simulink model "Push_pull_conv"  (R2021b)
settings: Solver=ode23s  StartTime=0.0  StopTime=inf  RelTol=1e-3
InitFcn:
  | % Target Load Voltage
  | v_ref = 48;
  | 
  | % Whether data should be broadcasted to Cloud / MQTT Ecosystem.
  | should_broadcast = true;
StartFcn:
  | if should_broadcast
  |     client = mqtt("tcp://rithviknishad.ddns.net");
  |     publish(client, "ps/state/IsRunning", "true");
  | end
StopFcn:
  | if should_broadcast
  |     client = mqtt("tcp://rithviknishad.ddns.net");
  |     publish(client, "ps/state/IsRunning", "false");
  | end
model workspace (MAT data in the model file):
  moreload = 1
undefined symbols (not defined in the file or in its folder): Ion, Lithium
libraries: spsSeriesRLCBranchLib x6, spsIdealSwitchLib x4, spsDiodeLib x4, spsMeanLib x3, simulink x3, spsCurrentMeasurementLib x2, spsGroundLib x2, spsMosfetLib x2, spsVariableResistorLib x1, slpidlib x1, spsPWMGeneratorDCDCLib x1, spsMultiWindingTransformerLib x1
(part 2 of 2)

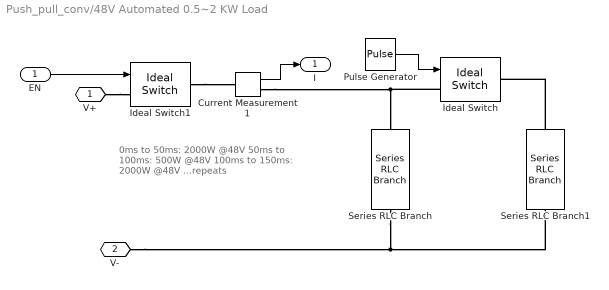
== system Push_pull_conv/48V Automated 0.5~2 KW Load ==
  note: 0ms to 50ms: 2000W @48V
      | 50ms to 100ms: 500W @48V
      | 100ms to 150ms: 2000W @48V
      | ...repeats
  EN : Inport
  Current Measurement1 : spsCurrentMeasurementLib/Current Measurement  PhasorSimulation=off  OutputType=Complex  PSBequivalent=0
  Ideal Switch : spsIdealSwitchLib/Ideal Switch  Ron=0.00000001  Lon=0  IC=0  Rs=1e5  Cs=inf  Measurements=off
  Ideal Switch1 : spsIdealSwitchLib/Ideal Switch  Ron=0.00000001  Lon=0  IC=0  Rs=1e5  Cs=inf  Measurements=off
  Pulse Generator : DiscretePulseGenerator  PulseType=Time based  Period=0.05  PulseWidth=50  PhaseDelay=0 * 0.1
  Series RLC Branch : spsSeriesRLCBranchLib/Series RLC Branch  LConnTagsString=__new0  RConnTagsString=__new0  BranchType=R  Resistance=48*48/500  Inductance=1e-3  SetiL0=off  InitialCurrent=0  Capacitance=41.42e-3  Setx0=off  InitialVoltage=0  Measurements=None
  Series RLC Branch1 : spsSeriesRLCBranchLib/Series RLC Branch  LConnTagsString=__new0  RConnTagsString=__new0  BranchType=R  Resistance=48*48/1500  Inductance=1e-3  SetiL0=off  InitialCurrent=0  Capacitance=41.42e-3  Setx0=off  InitialVoltage=0  Measurements=None
  V+ : PMIOPort  Side=Left
  V- : PMIOPort  Port=2  Side=Right
  I : Outport
  wires:
  Current Measurement1/1 -> I/1
  Pulse Generator/1 -> Ideal Switch/1
  EN/1 -> Ideal Switch1/1
  connections:
  Ideal Switch/LConn1 -- Series RLC Branch/LConn1 -- Current Measurement1/RConn1
  Series RLC Branch1/LConn1 -- Ideal Switch/RConn1
  Ideal Switch1/RConn1 -- Current Measurement1/LConn1
  Series RLC Branch1/RConn1 -- V-/RConn1 -- Series RLC Branch/RConn1
  V+/RConn1 -- Ideal Switch1/LConn1

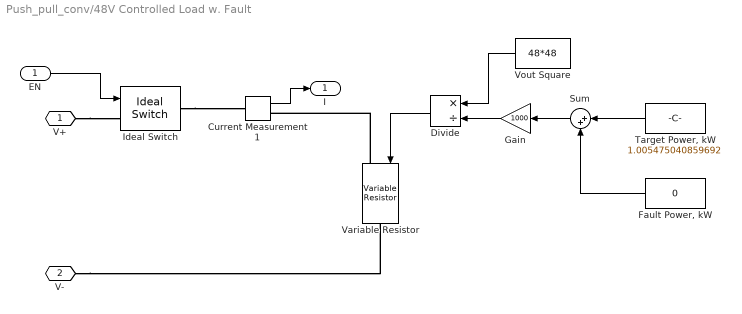
== system Push_pull_conv/48V Controlled Load w. Fault ==
  EN : Inport
  Current Measurement1 : spsCurrentMeasurementLib/Current Measurement  PhasorSimulation=off  OutputType=Complex  PSBequivalent=0
  Divide : Product  Inputs=*/
  "Fault Power, kW" : Constant  Value=0
  Gain : Gain  Gain=1000
  Ideal Switch : spsIdealSwitchLib/Ideal Switch  Ron=0.00000001  Lon=0  IC=0  Rs=1e5  Cs=inf  Measurements=off
  Sum : Sum  Inputs=|++
  "Target Power, kW" : Constant  Value=1.005475040859692
  Variable Resistor : spsVariableResistorLib/Variable Resistor  Rabsmin=1e-3
      settings: SourceProductBaseCode=PS
  Vout Square : Constant  Value=48*48
  V+ : PMIOPort  Side=Left
  V- : PMIOPort  Port=2  Side=Right
  I : Outport
  wires:
  Current Measurement1/1 -> I/1
  Vout Square/1 -> Divide/1
  Divide/1 -> Variable Resistor/1
  Gain/1 -> Divide/2
  EN/1 -> Ideal Switch/1
  "Target Power, kW"/1 -> Sum/1
  Sum/1 -> Gain/1
  "Fault Power, kW"/1 -> Sum/2
  connections:
  Ideal Switch/RConn1 -- Current Measurement1/LConn1
  Variable Resistor/LConn1 -- Current Measurement1/RConn1
  V+/RConn1 -- Ideal Switch/LConn1
  V-/RConn1 -- Variable Resistor/RConn1

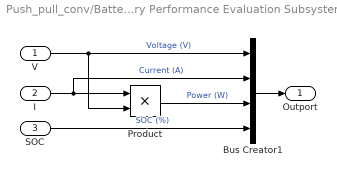
== system Push_pull_conv/Battery Performance Evaluation Subsystem ==
  V : Inport
  I : Inport  Port=2
  SOC : Inport  Port=3
  Bus Creator1 : BusCreator  Inputs=4
  Product : Product
  Outport : Outport
  wires:
  Bus Creator1/1 -> Outport/1
  I/1 -> Product/1, Bus Creator1/2  "Current (A)"
  V/1 -> Product/2, Bus Creator1/1  "Voltage (V)"
  Product/1 -> Bus Creator1/3  "Power (W)"
  SOC/1 -> Bus Creator1/4  "SOC (%)"

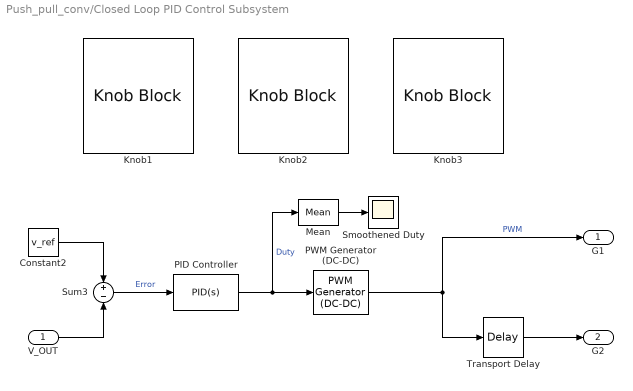
== system Push_pull_conv/Closed Loop PID Control Subsystem ==
  V_OUT : Inport
  Constant2 : Constant  Value=v_ref
  Knob1 : KnobBlock  LabelPosition=Bottom  ScaleMax=1  TickInterval=0.1
  Knob2 : KnobBlock  LabelPosition=Bottom  ScaleMax=1  TickInterval=0.1
  Knob3 : KnobBlock  LabelPosition=Bottom  ScaleMax=1  TickInterval=0.1
  Mean : spsMeanLib/Mean  Freq=150  Vinit=0  Ts=0
  PID Controller : slpidlib/PID Controller  Controller=PID  Form=Parallel  TimeDomain=Continuous-time  UseExternalTs=off  SampleTime=-1  IntegratorMethod=Forward Euler  FilterMethod=Forward Euler  ControllerParametersSource=internal  P=0.1  I=0.1  D=0  UseFilter=on  N=100  TunerSelectOption=Transfer Function Based (PID Tuner App)  InitialConditionSource=internal  InitialConditionForIntegrator=0  InitialConditionForFilter=0  DifferentiatorICPrevScaledInput=0  ExternalReset=none  TrackingMode=off  Kt=1  LimitOutput=on  SatLimitsSource=internal  UpperSaturationLimit=0.5  LowerSaturationLimit=0  LinearizeAsGain=off  AntiWindupMode=none  Kb=1  POutMin=[]  POutMax=[]  IOutMin=[]  IOutMax=[]  DOutMin=[]  DOutMax=[]  NOutMin=[]  NOutMax=[]  SumOutMin=[]  SumOutMax=[]  SaturationOutMin=[]  SaturationOutMax=[]  PParamMin=[]  PParamMax=[]  IParamMin=[]  IParamMax=[]  DParamMin=[]  DParamMax=[]  NParamMin=[]  NParamMax=[]  KbParamMin=[]  KbParamMax=[]  KtParamMin=[]  KtParamMax=[]  KbOutMin=[]  KbOutMax=[]  KtOutMin=[]  KtOutMax=[]  IntegratorOutMin=[]  IntegratorOutMax=[]  FilterOutMin=[]  FilterOutMax=[]  SumI1OutMin=[]  SumI1OutMax=[]  SumI2OutMin=[]  SumI2OutMax=[]  SumI3OutMin=[]  SumI3OutMax=[]  SumI4OutMin=[]  SumI4OutMax=[]  SumDOutMin=[]  SumDOutMax=[]  DifferentiatorOutMin=[]  DifferentiatorOutMax=[]  FilterDiffOutCoefMin=[]  FilterDiffOutCoefMax=[]  ReciprocalOutMin=[]  ReciprocalOutMax=[]  SumDenOutMin=[]  SumDenOutMax=[]  SumNumOutMin=[]  SumNumOutMax=[]  DivideOutMin=[]  DivideOutMax=[]  UdiffTsProdOutMin=[]  UdiffTsProdOutMax=[]  NTsProdOutMin=[]  NTsProdOutMax=[]  UintegralTsProdOutMin=[]  UintegralTsProdOutMax=[]  UngainTsProdOutMin=[]  UngainTsProdOutMax=[]  IntegratorContinuousStateAttributes=''  IntegratorStateMustResolveToSignalObject=off  IntegratorRTWStateStorageClass=Auto  FilterContinuousStateAttributes=''  FilterStateMustResolveToSignalObject=off  FilterRTWStateStorageClass=Auto  ParallelPVariant=InternalParameters  IdealPVariant=Disabled  IVariant=InternalParameters  DVariant=InternalParameters  IntegratorVariant=Continuous  SatVariant=Enabled  AWVariant=Passthrough  PCopyVariant=Disabled  TRVariant=Disabled  FdbkBlocksVariant=Forward  IdealPFdbkVariant=Disabled  SatFdbkVariant=Disabled  DerivativeFilterVariant=ContFilter  NVariant=InternalParameters  NCopyVariant=Disabled  FilterICVariant=InternalICsFilter  IntegratorICVariant=InternalICs  ExternalResetVariant=Disabled  TRSumVariant=Passthrough  SumFdbkVariant=Disabled  SumVariant=Sum_PID  TsampFilterVariant=InternalTs  TsampNgainVariant=Passthrough  TsampIntegralVariant=Passthrough  ExternalSaturationOutDataTypeStr=Inherit: Same as second input
  PWM Generator (DC-DC) : spsPWMGeneratorDCDCLib/PWM Generator (DC-DC)  Fsw=150e3  Ts=0
  Smoothened Duty : Scope
  Sum3 : Sum  Inputs=+-
  Transport Delay : TransportDelay  DelayTime=180/(360*150e3)
  G1 : Outport
  G2 : Outport  Port=2
  wires:
  Constant2/1 -> Sum3/1
  V_OUT/1 -> Sum3/2
  PWM Generator (DC-DC)/1 -> G1/1, Transport Delay/1  "PWM"
  Sum3/1 -> PID Controller/1  "Error"
  PID Controller/1 -> Mean/1, PWM Generator (DC-DC)/1  "Duty"
  Mean/1 -> Smoothened Duty/1
  Transport Delay/1 -> G2/1

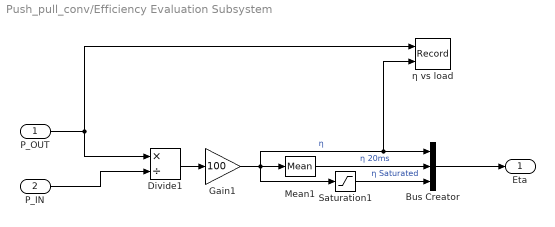
== system Push_pull_conv/Efficiency Evaluation Subsystem ==
  P_OUT : Inport
  P_IN : Inport  Port=2
  Bus Creator : BusCreator  Inputs=3
  Divide1 : Product  Inputs=*/
  Gain1 : Gain  Gain=100
  Mean1 : spsMeanLib/Mean  Freq=50  Vinit=0  Ts=0
  Saturation1 : Saturate  UpperLimit=100
  η vs load : Record  FileSettingsInternal="{\"entries\":[{\"content\":{\"excelSettings\":{\"content\":{},\"type\":\"Streamout.ExcelSettings\"}},\"type\":\"Streamout.FileSettingStorage\",\"uuid\":\"d06f74cc-fced-4a1e-9c31-17602b41e559\"}],\"packageUris\":[\"http://schema.mathworks.com/mf0/streamout_blocks/R2020a\"],\"version\":\"1.0\"}"  Layout=[1 1]  SignalsInternal="{\"entries\":[{\"content\":{\"signals\":[{\"content\":{\"blockPath\":[\"Push_pull_conv/Efficiency Evaluation Subsystem/η vs load\"],\"channel\":[],\"dimensions\":[1],\"domain\":\"Push_pull_conv/Efficiency Evaluation Subsystem/ￎﾷ vs load\",\"lineColor\":\"#64d413\",\"plots\":[],\"port\":1,\"sid\":[\"\"],\"signalID\":227180,\"signalName\":\"P_OUT\"},\"type\":\"RecordBlkView.Signal\",\"uuid\":\"f3186113-8e68-4c99-bf8f-1509c4a87657\"},{\"content\":{\"blockPath\":[\"Push_pull_conv/Efficiency Evaluation Subsystem/η vs load\"],\"channel\":[],\"dimensions\":[1],\"domain\":\"Push_pull_conv/Efficiency Evaluation Subsystem/ￎﾷ vs load\",\"lineColor\":\"#ff13a6\",\"plots\":[],\"port\":2,\"sid\":[\"\"],\"signalID\":227184,\"signalName\":\"η\"},\"type\":\"RecordBlkView.Signal\",\"uuid\":\"933036bb-5959-4669-957e-8a4b6c9fc7ee\"}]},\"type\":\"RecordBlkView.InputSignals\",\"uuid\":\"264eb576-88f5-4594-8ef1-38e7c656bcfb\"}],\"packageUris\":[\"http://schema.mathworks.com/mf0/streamout_blocks/R2020a\"],\"version\":\"1.0\"}"  VisualizationBindings="{\"xyplotplugin\":{\"info\":[{\"series\":[],\"subplotID\":1}]}}"  CompatibilityTag=XY
  Eta : Outport
  wires:
  Gain1/1 -> Saturation1/1, η vs load/2, Bus Creator/1, Mean1/1  "η"
  Saturation1/1 -> Bus Creator/3  "η Saturated"
  Divide1/1 -> Gain1/1
  Mean1/1 -> Bus Creator/2  "η 20ms"
  Bus Creator/1 -> Eta/1
  P_IN/1 -> Divide1/2
  P_OUT/1 -> η vs load/1, Divide1/1

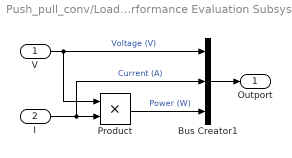
== system Push_pull_conv/Load Performance Evaluation Subsystem ==
  V : Inport
  I : Inport  Port=2
  Bus Creator1 : BusCreator  Inputs=3
  Product : Product
  Outport : Outport
  wires:
  Bus Creator1/1 -> Outport/1
  I/1 -> Product/2, Bus Creator1/2  "Current (A)"
  V/1 -> Bus Creator1/1, Product/1  "Voltage (V)"
  Product/1 -> Bus Creator1/3  "Power (W)"

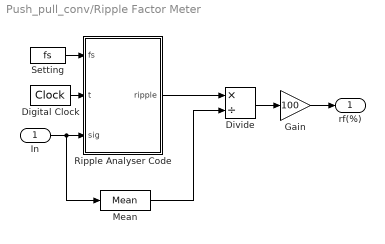
== system Push_pull_conv/Ripple Factor Meter ==
  In : Inport
  Digital Clock : DigitalClock  SampleTime=1/fs/Nsam
  Divide : Product  Inputs=*/
  Gain : Gain  Gain=100
  Mean : spsMeanLib/Mean  Freq=fs  Vinit=0  Ts=0
  Ripple Analyser Code : MATLAB Function  TreatAsAtomicUnit=on  SystemSampleTime=1/fs/Nsam
  Setting : Constant  Value=fs
  rf(%) : Outport
  wires:
  Ripple Analyser Code/1(ripple) -> Divide/1
  Mean/1 -> Divide/2
  Setting/1 -> Ripple Analyser Code/1(fs)
  Digital Clock/1 -> Ripple Analyser Code/2(t)
  In/1 -> Mean/1, Ripple Analyser Code/3(sig)
  Divide/1 -> Gain/1
  Gain/1 -> rf(%)/1

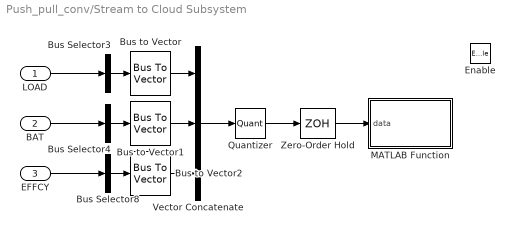
== system Push_pull_conv/Stream to Cloud Subsystem ==
  LOAD : Inport
  BAT : Inport  Port=2
  EFFCY : Inport  Port=3
  Enable : EnablePort
  Bus Selector3 : BusSelector  OutputSignals=Voltage (V),Current (A),Power (W)  OutputAsBus=on
  Bus Selector4 : BusSelector  OutputSignals=Voltage (V),Current (A),Power (W)  OutputAsBus=on
  Bus Selector8 : BusSelector  OutputSignals=η  OutputAsBus=on
  Bus to Vector : BusToVector
  Bus to Vector1 : BusToVector
  Bus to Vector2 : BusToVector
  MATLAB Function : MATLAB Function  TreatAsAtomicUnit=on  SystemSampleTime=0.001
  Quantizer : Quantizer  QuantizationInterval=0.1
  Vector Concatenate : Concatenate  NumInputs=3
  Zero-Order Hold : ZeroOrderHold  SampleTime=-1
  wires:
  Vector Concatenate/1 -> Quantizer/1
  LOAD/1 -> Bus Selector3/1
  Bus to Vector1/1 -> Vector Concatenate/2
  BAT/1 -> Bus Selector4/1
  Bus to Vector/1 -> Vector Concatenate/1
  Zero-Order Hold/1 -> MATLAB Function/1(data)
  Bus Selector3/1 -> Bus to Vector/1
  Bus Selector4/1 -> Bus to Vector1/1
  Bus Selector8/1 -> Bus to Vector2/1
  Quantizer/1 -> Zero-Order Hold/1
  EFFCY/1 -> Bus Selector8/1
  Bus to Vector2/1 -> Vector Concatenate/3

== matlab function Push_pull_conv/Ripple Factor Meter/Ripple Analyser Code ==
  data: fs input; t input; sig input; ripple output
function ripple  = ripAnaly(fs,t,sig)
%% Create Memory
persistent m
if isempty(m)
	m.min = inf;
	m.max = -inf;
    m.riph = 0;
end

%% Min-Max Updater
if m.min>sig
    m.min=sig;
end
if m.max<sig
    m.max=sig;
end

%% Reset Timer
Phase=rem(t,1/fs)*fs;
if Phase==0
    rip=m.max-m.min;
    m.riph=rip;
    m.min = inf;
	m.max = -inf;
end
ripple=m.riph;

== matlab function Push_pull_conv/Stream to Cloud Subsystem/MATLAB Function ==
  data: data input
function pub_to_mqtt(data)

    % Referred from: https://blogs.mathworks.com/simulink/2014/01/08/simulink-and-matlab-objects/
    coder.extrinsic('iot_ppc_broadcast_to_mqtt');

    % Propogate `data` and invoke the extrinsic function.
    iot_ppc_broadcast_to_mqtt(data)
end
